simulink model "id_model"  (R2019b)
settings: Solver=VariableStepAuto  StartTime=0.0  StopTime=100  RelTol=1e-3
values from neighbouring files (symbols this model uses):
  Alat = [-0.1180 32.033 0 0 ... (first row only)    [model.m]
  Blat = [0 ... (first row only)    [model.m]
  Clat = [0.3048 0 0 0]    [model.m]
undefined symbols (not defined in the file or in its folder): DEN, DENL, NUM, NUML
settings Model: Creator=Merc  LastModifiedBy=brian
settings DataIOCC: ReturnWorkspaceOutputs=off
settings DebuggingCC: ArithmeticOperatorsInVariantConditions=warning
settings SFSimCC: CustomCodeUndefinedFunction=UseInterfaceOnly

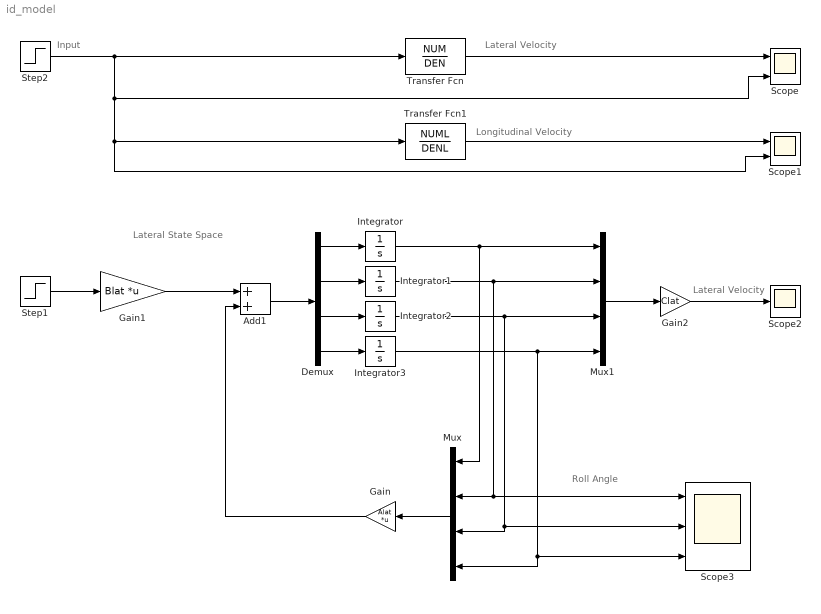
== system id_model ==
  note: Lateral State Space
  note: Lateral Velocity
  note: Roll Angle
  note: Longitudinal Velocity
  note: Input
  note: Lateral Velocity
  Add1 : Sum
  Demux : Demux
  Gain : Gain  Gain=Alat  Multiplication=Matrix(K*u)
  Gain1 : Gain  Gain=Blat  Multiplication=Matrix(K*u)
  Gain2 : Gain  Gain=Clat
  Integrator{,1..3} (4 alike) : Integrator
  Mux : Mux
  Mux1 : Mux
  Scope : Scope  NumInputPorts=2
  Scope1 : Scope  NumInputPorts=2
  Scope2 : Scope
  Scope3 : Scope  NumInputPorts=3
  Step1 : Step  After=0.5  SampleTime=0
  Step2 : Step  After=1500  SampleTime=0
  Transfer Fcn : TransferFcn  Numerator=NUM  Denominator=DEN
  Transfer Fcn1 : TransferFcn  Numerator=NUML  Denominator=DENL
  wires:
  Step2/1 -> Transfer Fcn/1, Scope1/2, Transfer Fcn1/1, Scope/2
  Transfer Fcn1/1 -> Scope1/1
  Transfer Fcn/1 -> Scope/1
  Mux/1 -> Gain/1
  Integrator/1 -> Mux/1, Mux1/1
  Integrator1/1 -> Scope3/1, Mux/2, Mux1/2
  Integrator2/1 -> Mux1/3, Scope3/2, Mux/3
  Integrator3/1 -> Mux/4, Scope3/3, Mux1/4
  Gain/1 -> Add1/2
  Gain1/1 -> Add1/1
  Demux/1 -> Integrator/1
  Demux/2 -> Integrator1/1
  Demux/3 -> Integrator2/1
  Demux/4 -> Integrator3/1
  Step1/1 -> Gain1/1
  Gain2/1 -> Scope2/1
  Add1/1 -> Demux/1
  Mux1/1 -> Gain2/1
